simulink subsystem "startComputeQuaternionError"  (R2021a)
settings: Solver=VariableStepAuto  StartTime=0.0  StopTime=10.0  RelTol=1e-3
settings Model: Creator=noraw  LastModifiedBy=noraw

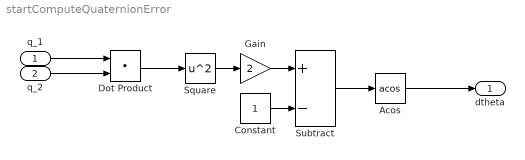
== system startComputeQuaternionError ==
  q_1 : Inport
  q_2 : Inport  Port=2
  Acos : Trigonometry  Operator=acos
  Constant : Constant
  Dot Product : DotProduct  InputSameDT=on  OutDataTypeStr=Inherit: Inherit via internal rule
  Gain : Gain  Gain=2
  Square : Math  Operator=square  SaturateOnIntegerOverflow=on
  Subtract : Sum  Inputs=+-
  dtheta : Outport
  wires:
  Square/1 -> Gain/1
  Dot Product/1 -> Square/1
  Acos/1 -> dtheta/1
  Gain/1 -> Subtract/1
  q_1/1 -> Dot Product/1
  Subtract/1 -> Acos/1
  Constant/1 -> Subtract/2
  q_2/1 -> Dot Product/2
